simulink model "RM35"
settings: Solver=ode4  StartTime=0  StopTime=400  FixedStep=0.1  RelTol=1e-3  EnableMultiTasking=on
undefined symbols (not defined in the file): body, constraint, pto
libraries: WECSim_Lib x5

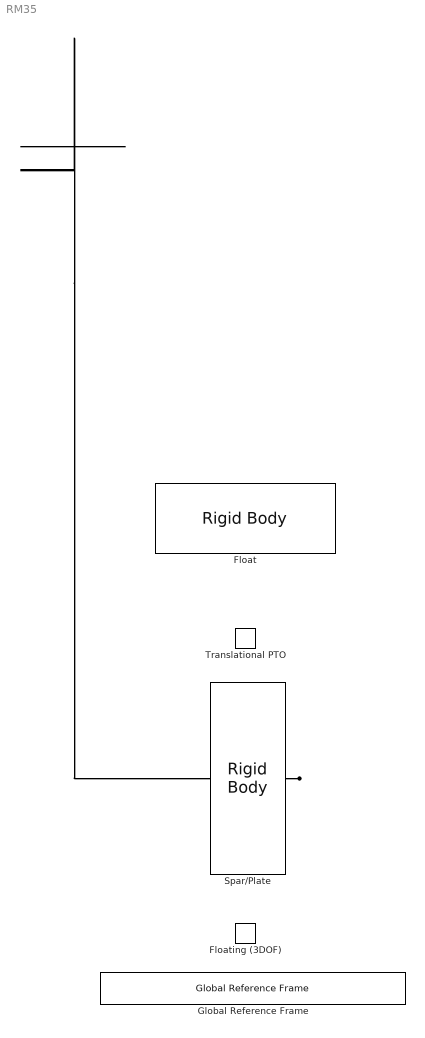
== system RM35 ==
  Float : WECSim_Lib/Body Elements/Rigid Body  body=body(1)  body=body(1)  body=body(1)  body=body(1)
      settings: AttributesFormatString=%<body>
  Floating (3DOF) : WECSim_Lib/Constraints/Floating (3DOF)  constraint=constraint(1)  constraint=constraint(1)  constraint=constraint(1)  constraint=constraint(1)
      settings: AttributesFormatString=%<constraint>
  Global Reference Frame : WECSim_Lib/Frames/Global Reference Frame  waves=waves  simu=simu  waves=waves  simu=simu  waves=waves  simu=simu  waves=waves  simu=simu
  Spar/Plate : WECSim_Lib/Body Elements/Rigid Body  body=body(2)  body=body(2)  body=body(2)  body=body(2)
      settings: AttributesFormatString=%<body>
  Translational PTO : WECSim_Lib/PTOs/Translational PTO  pto=pto(1)  pto=pto(1)  pto=pto(1)  pto=pto(1)
      settings: AttributesFormatString=%<pto>
  connections:
  ?
  ?
  ?
